simulink model "waterTankBurner"  (R2014b)
settings: Solver=FixedStepDiscrete  StartTime=0.0  StopTime=100000  FixedStep=0.01  MaxStep=0.0001  RelTol=1e-3
settings Model: Creator=sand080  LastModifiedBy=sand080
settings DataIOCC: LimitDataPoints=off

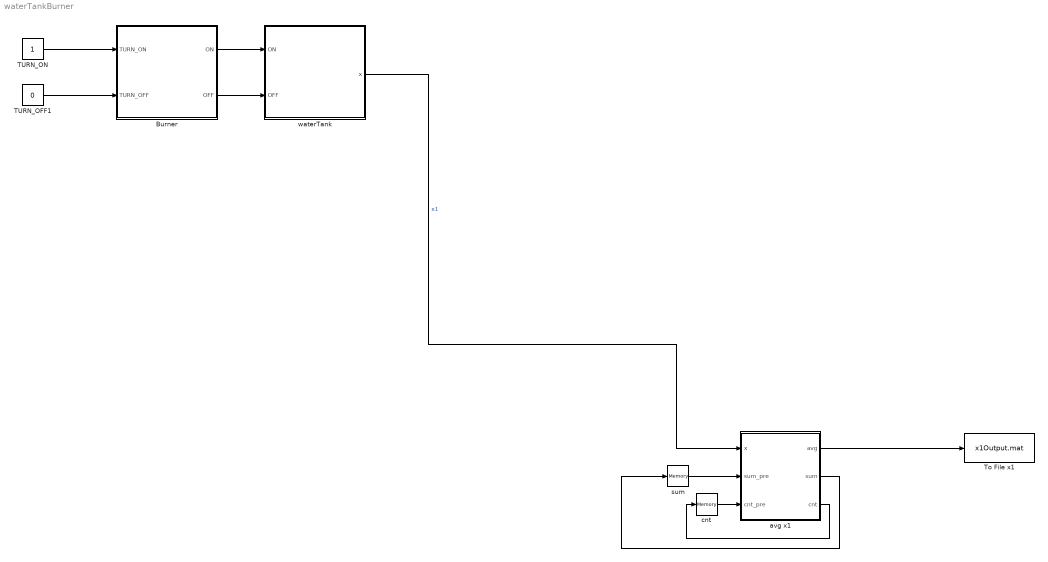
== system waterTankBurner ==
  Burner : Subsystem
  TURN_OFF1 : Constant  Value=0
  TURN_ON : Constant
  To File x1 : ToFile  Filename=x1Output.mat
      settings: Decimation=10000000
  avg x1 : MATLAB Function  TreatAsAtomicUnit=on
  cnt : Memory
  sum : Memory
  waterTank : Subsystem
  wires:
  TURN_ON/1 -> Burner/1(TURN_ON)
  Burner/1(ON) -> waterTank/1(ON)
  Burner/2(OFF) -> waterTank/2(OFF)
  TURN_OFF1/1 -> Burner/2(TURN_OFF)
  waterTank/1(x) -> avg x1/1(x)  "x1"
  avg x1/2(sum) -> sum/1
  avg x1/3(cnt) -> cnt/1
  cnt/1 -> avg x1/3(cnt_pre)
  sum/1 -> avg x1/2(sum_pre)
  avg x1/1(avg) -> To File x1/1

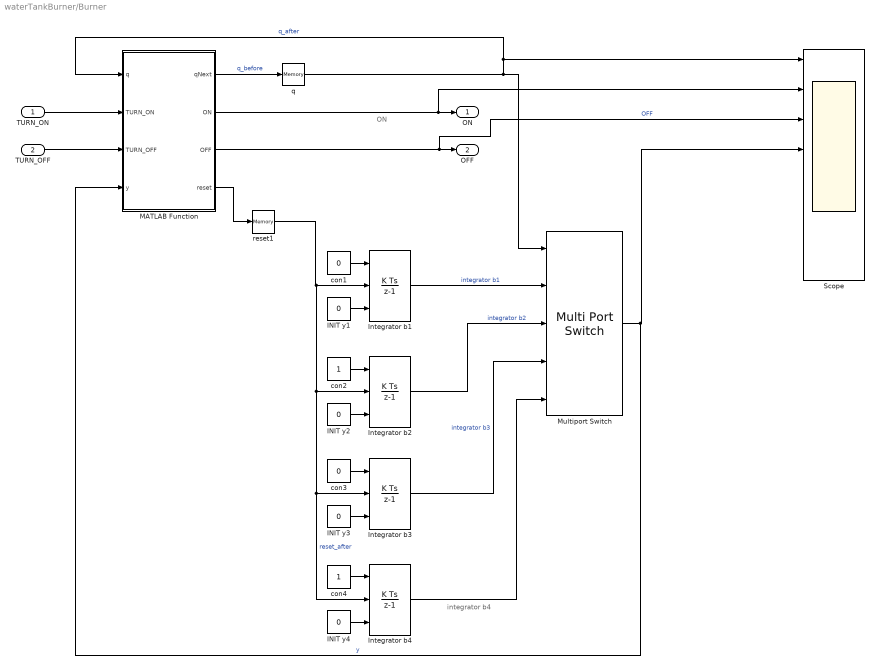
== system waterTankBurner/Burner ==
  note: integrator b4
  note: ON
  TURN_ON : Inport
  TURN_OFF : Inport  Port=2
  INIT y{1..4} (4 alike) : Constant  Value=0
  Integrator b{1..4} (4 alike) : DiscreteIntegrator  ExternalReset=either  InitialConditionSource=external  InitialCondition=510  InitialConditionSetting=State (most efficient)  SampleTime=-1
  MATLAB Function : MATLAB Function  Priority=1  TreatAsAtomicUnit=on
  Multiport Switch : MultiPortSwitch  Inputs=4
  Scope : Scope  NumInputPorts=8
      settings: TickLabels=on  ShowLegends=on  YMin=0~0~0~0~0~0~0~0  YMax=1~1~1~1~1~1~1~1
  con1 : Constant  Value=0
  con2 : Constant
  con3 : Constant  Value=0
  con4 : Constant
  q : Memory  X0=1  LinearizeMemory=on
  reset1 : Memory  LinearizeMemory=on
  ON : Outport
  OFF : Outport  Port=2
  wires:
  MATLAB Function/3(OFF) -> Scope/3, OFF/1  "OFF"
  INIT y1/1 -> Integrator b1/3
  INIT y2/1 -> Integrator b2/3
  con1/1 -> Integrator b1/1
  MATLAB Function/1(qNext) -> q/1  "q_before"
  q/1 -> Multiport Switch/1, MATLAB Function/1(q), Scope/1  "q_after"
  MATLAB Function/4(reset) -> reset1/1
  con2/1 -> Integrator b2/1
  MATLAB Function/2(ON) -> Scope/2, ON/1
  TURN_OFF/1 -> MATLAB Function/3(TURN_OFF)
  TURN_ON/1 -> MATLAB Function/2(TURN_ON)
  INIT y3/1 -> Integrator b3/3
  INIT y4/1 -> Integrator b4/3
  con3/1 -> Integrator b3/1
  con4/1 -> Integrator b4/1
  reset1/1 -> Integrator b4/2, Integrator b3/2, Integrator b2/2, Integrator b1/2  "reset_after"
  Integrator b1/1 -> Multiport Switch/2  "integrator b1"
  Integrator b2/1 -> Multiport Switch/3  "integrator b2"
  Integrator b3/1 -> Multiport Switch/4  "integrator b3"
  Integrator b4/1 -> Multiport Switch/5
  Multiport Switch/1 -> MATLAB Function/4(y), Scope/4  "y"

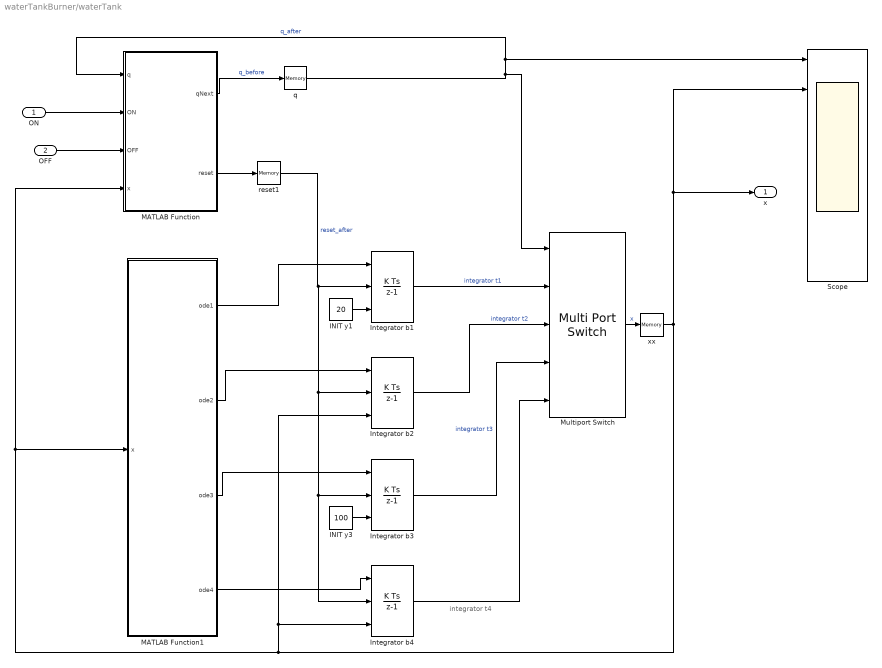
== system waterTankBurner/waterTank ==
  note: integrator t4
  ON : Inport
  OFF : Inport  Port=2
  INIT y1 : Constant  Value=20
  INIT y3 : Constant  Value=100
  Integrator b{1..4} (4 alike) : DiscreteIntegrator  ExternalReset=either  InitialConditionSource=external  InitialCondition=510  InitialConditionSetting=State (most efficient)  SampleTime=-1
  MATLAB Function : MATLAB Function  Priority=1  TreatAsAtomicUnit=on
  MATLAB Function1 : MATLAB Function  TreatAsAtomicUnit=on
  Multiport Switch : MultiPortSwitch  Inputs=4
  Scope : Scope  NumInputPorts=8
      settings: TickLabels=on  ShowLegends=on  YMin=0~0~0~0~0~0~0~0  YMax=1~1~1~1~1~1~1~1
  q : Memory  X0=1  LinearizeMemory=on
  reset1 : Memory  LinearizeMemory=on
  xx : Memory  LinearizeMemory=on
  x : Outport
  wires:
  INIT y1/1 -> Integrator b1/3
  MATLAB Function1/1(ode1) -> Integrator b1/1
  MATLAB Function/1(qNext) -> q/1  "q_before"
  q/1 -> Multiport Switch/1, MATLAB Function/1(q), Scope/1  "q_after"
  MATLAB Function/2(reset) -> reset1/1
  MATLAB Function1/2(ode2) -> Integrator b2/1
  INIT y3/1 -> Integrator b3/3
  MATLAB Function1/3(ode3) -> Integrator b3/1
  MATLAB Function1/4(ode4) -> Integrator b4/1
  reset1/1 -> Integrator b4/2, Integrator b3/2, Integrator b2/2, Integrator b1/2  "reset_after"
  Integrator b1/1 -> Multiport Switch/2  "integrator t1"
  Integrator b2/1 -> Multiport Switch/3  "integrator t2"
  Integrator b3/1 -> Multiport Switch/4  "integrator t3"
  Integrator b4/1 -> Multiport Switch/5
  OFF/1 -> MATLAB Function/3(OFF)
  ON/1 -> MATLAB Function/2(ON)
  xx/1 -> x/1, Scope/2, Integrator b2/3, Integrator b4/3, MATLAB Function1/1(x), MATLAB Function/4(x)
  Multiport Switch/1 -> xx/1  "x"

== matlab function waterTankBurner/waterTank/MATLAB Function ==
  data: q input; ON input; OFF input; x input; qNext output; reset output


function [qNext,reset]  = phi(q,  ON, OFF,x)
%#codegen


if q==1 % q=1, tank is in t1
    if ON==0
        qNext=1;
        reset=0;
    elseif ON==1
        qNext=2;
        reset=1;
    else
        qNext=-1;
        reset=-1;
    end;
    
elseif q==2 % q=2, tank is in t2
    if x<100 && OFF==0
        qNext=2;
        reset=0;
    elseif x>=100
        qNext=3;
        reset=1;
    elseif x<100 && OFF==1
        qNext=4;
        reset=1;
    else
        qNext=-1;
        reset=-1;
    end;

elseif q==3 % q=3, tank is in state t3
    if OFF==0
        qNext=3;
        reset=0;
    elseif OFF==1
        qNext=4;
        reset=1;
    else
        qNext=-1;
        reset=-1;
    end;
elseif q==4 % q=4, tank is in state t4
    if x>20 && ON==0
        qNext=4;
        reset=0;
    elseif x<=20
        qNext=1;
        reset=1;
    elseif x>20 && ON==1
        qNext=2;
        reset=1;
    else
        qNext=-1;
        reset=-1;
    end;
else
    qNext=-1; %this should never execute
    reset=-1;%this should never execute
end

== matlab function waterTankBurner/Burner/MATLAB Function ==
  data: q input; TURN_ON input; TURN_OFF input; qNext output; ON output; OFF output; y input; reset output


function [qNext,ON,OFF,reset]  = phi(q,  TURN_ON, TURN_OFF,y)
%#codegen


if q==1 % q=1, burner is in state b1
    if TURN_ON==0
        qNext=1;
        reset=0;
        ON=0;
        OFF=0;
    elseif TURN_ON==1
        qNext=2;
        reset=1;
        ON=0;
        OFF=0;
    else
        qNext=-1;
        reset=-1;
        ON=-1;
        OFF=-1;
    end;
    
elseif q==2 % q=2, burner is in state b2
    if y>= 0.1
        qNext=3;
        reset=1;
        ON=1;
        OFF=0;
    elseif y< 0.1
        qNext=2;
        reset=0;
        ON=0;
        OFF=0;
    else
        qNext=-1;
        reset=-1;
        ON=-1;
        OFF=-1;
    end;

elseif q==3 % q=3, burner is in state b3
    if TURN_OFF==0
        qNext=3;
        reset=0;
        ON=0;
        OFF=0;
    elseif TURN_OFF==1
        qNext=4;
        reset=1;
        ON=0;
        OFF=0;
    else
        qNext=-1;
        reset=-1;
        ON=-1;
        OFF=-1;
    end;
elseif q==4 % q=4, burner is in state b4
    if y< 0.1
        qNext=4;
        reset=0;
        ON=0;
        OFF=0;
    elseif y>= 0.1
        qNext=1;
        reset=1;
        ON=0;
        OFF=1;
    else
        qNext=-1;
        reset=-1;
        ON=-1;
        OFF=-1;
    end;
else
    qNext=-1; %this should never execute
    reset=-1;%this should never execute
    ON=-1;%this should never execute
    OFF=-1;%this should never execute
    qNext=-1; %this should never execute
end

== matlab function waterTankBurner/waterTank/MATLAB Function1 ==
  data: x input; ode1 output; ode2 output; ode3 output; ode4 output
function [ode1,ode2,ode3,ode4] = ODEs(x)
%#codegen
K=0.075;
h=150;
ode1=0;
ode2=K*(h-x);
ode3=0;
ode4=-K*x;

== matlab function waterTankBurner/avg x1 ==
  data: x input; avg output; sum output; cnt output; sum_pre input; cnt_pre input
function [avg, sum,cnt] = fcn(x,  sum_pre, cnt_pre)
%#codegen

cnt=cnt_pre+1;
sum=sum_pre+x;
avg=sum/cnt;
